simulink model "hpt_dual_dcpool_sw"  (R2025a)
settings: Solver=ode23tb  StartTime=0.0  StopTime=0.5  RelTol=1e-3
libraries: spsSeriesRLCBranchLib x5, spsControlledCurrentSourceLib x2, spsThreePhaseSeriesRLCBranchLib x2, spsThreePhaseVIMeasurementLib x2, spsVoltageMeasurementLib x2, spsUniversalBridgeLib x2, spsThreePhaseSourceLib x2, spsGroundLib x1, spsCurrentMeasurementLib x1, spspowerguiLib x1
settings Model: Creator=m1391  LastModifiedBy=m1391

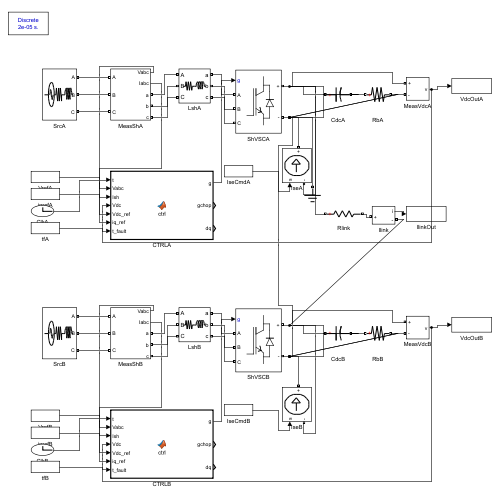
[thumbnail: Simulink's stored preview of the top-level diagram]
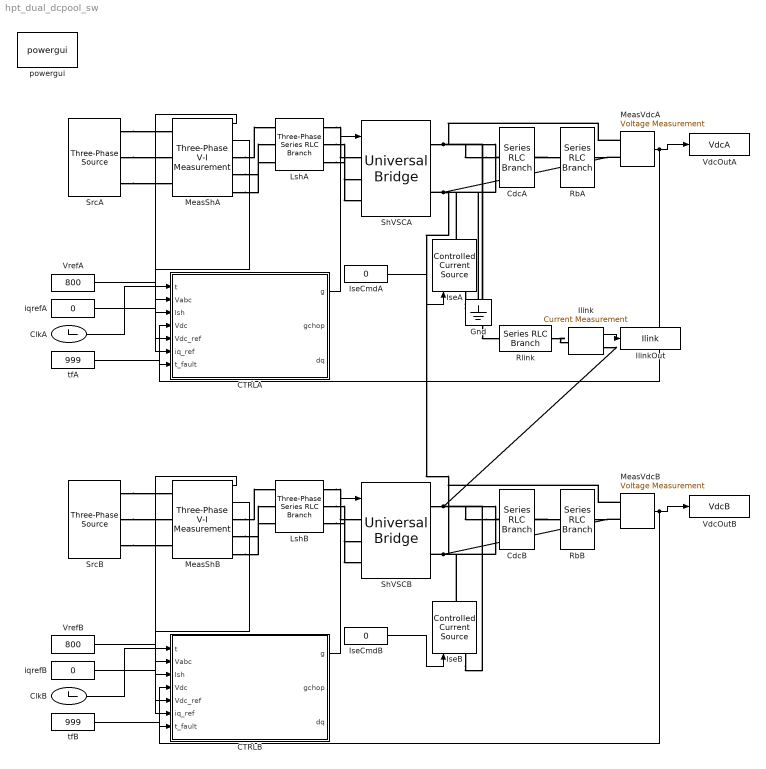
== system hpt_dual_dcpool_sw ==
  CTRLA : MATLAB Function  TreatAsAtomicUnit=on
  CTRLB : MATLAB Function  TreatAsAtomicUnit=on
  CdcA : spsSeriesRLCBranchLib/Series RLC Branch  LConnTagsString=__new0  RConnTagsString=__new0  BranchType=C  Resistance=1  Inductance=1e-3  SetiL0=off  InitialCurrent=0  Capacitance=0.0022  Setx0=on  InitialVoltage=800  Measurements=None
  CdcB : spsSeriesRLCBranchLib/Series RLC Branch  LConnTagsString=__new0  RConnTagsString=__new0  BranchType=C  Resistance=1  Inductance=1e-3  SetiL0=off  InitialCurrent=0  Capacitance=0.0022  Setx0=on  InitialVoltage=800  Measurements=None
  ClkA : Clock
  ClkB : Clock
  Gnd : spsGroundLib/Ground  LConnTagsString=a
  Ilink : spsCurrentMeasurementLib/Current Measurement  PhasorSimulation=off  OutputType=Complex  PSBequivalent=0
  IlinkOut : ToWorkspace  VariableName=Ilink  SampleTime=2e-05
  IseA : spsControlledCurrentSourceLib/Controlled Current Source  Initialize=on  Source_Type=AC  Amplitude=0  Phase=0  Frequency=0  Measurements=None
  IseB : spsControlledCurrentSourceLib/Controlled Current Source  Initialize=on  Source_Type=AC  Amplitude=0  Phase=0  Frequency=0  Measurements=None
  IseCmdA : Constant  Value=0
  IseCmdB : Constant  Value=0
  LshA : spsThreePhaseSeriesRLCBranchLib/Three-Phase Series RLC Branch  LConnTagsString=A|B|C  RConnTagsString=A|B|C  BranchType=RL  Resistance=0.05  Inductance=0.003  Capacitance=1e-6  Measurements=None
  LshB : spsThreePhaseSeriesRLCBranchLib/Three-Phase Series RLC Branch  LConnTagsString=A|B|C  RConnTagsString=A|B|C  BranchType=RL  Resistance=0.05  Inductance=0.003  Capacitance=1e-6  Measurements=None
  MeasShA : spsThreePhaseVIMeasurementLib/Three-Phase V-I Measurement  VoltageMeasurement=phase-to-ground  SetLabelV=off  LabelV=Vabc  Vpu=off  VpuLL=off  CurrentMeasurement=yes  SetLabelI=off  LabelI=Iabc  Ipu=off  Pbase=100e6  Vbase=500e3  OutputType=Complex  PhasorSimulation=off  PSBequivalent=0
  MeasShB : spsThreePhaseVIMeasurementLib/Three-Phase V-I Measurement  VoltageMeasurement=phase-to-ground  SetLabelV=off  LabelV=Vabc  Vpu=off  VpuLL=off  CurrentMeasurement=yes  SetLabelI=off  LabelI=Iabc  Ipu=off  Pbase=100e6  Vbase=500e3  OutputType=Complex  PhasorSimulation=off  PSBequivalent=0
  MeasVdcA : spsVoltageMeasurementLib/Voltage Measurement  PhasorSimulation=off  OutputType=Complex  PSBequivalent=0
  MeasVdcB : spsVoltageMeasurementLib/Voltage Measurement  PhasorSimulation=off  OutputType=Complex  PSBequivalent=0
  RbA : spsSeriesRLCBranchLib/Series RLC Branch  LConnTagsString=__new0  RConnTagsString=__new0  BranchType=R  Resistance=1e4  Inductance=1e-3  SetiL0=off  InitialCurrent=0  Capacitance=1e-6  Setx0=off  InitialVoltage=0  Measurements=None
  RbB : spsSeriesRLCBranchLib/Series RLC Branch  LConnTagsString=__new0  RConnTagsString=__new0  BranchType=R  Resistance=1e4  Inductance=1e-3  SetiL0=off  InitialCurrent=0  Capacitance=1e-6  Setx0=off  InitialVoltage=0  Measurements=None
  Rlink : spsSeriesRLCBranchLib/Series RLC Branch  LConnTagsString=__new0  RConnTagsString=__new0  BranchType=R  Resistance=0.5  Inductance=1e-3  SetiL0=off  InitialCurrent=0  Capacitance=1e-6  Setx0=off  InitialVoltage=0  Measurements=None
  ShVSCA : spsUniversalBridgeLib/Universal Bridge  Arms=3  SnubberResistance=1e5  SnubberCapacitance=inf  Device=IGBT / Diodes  Ron=1e-3  Lon=0  ForwardVoltages="[  0  0  ]"  ForwardVoltage=0  GTOparameters=[ 10e-6 , 20e-6 ]  IGBTparameters=[ 1e-6 , 2e-6 ]  Measurements=None  Measurements_2=None  converterType=Rectifier
  ShVSCB : spsUniversalBridgeLib/Universal Bridge  Arms=3  SnubberResistance=1e5  SnubberCapacitance=inf  Device=IGBT / Diodes  Ron=1e-3  Lon=0  ForwardVoltages="[  0  0  ]"  ForwardVoltage=0  GTOparameters=[ 10e-6 , 20e-6 ]  IGBTparameters=[ 1e-6 , 2e-6 ]  Measurements=None  Measurements_2=None  converterType=Rectifier
  SrcA : spsThreePhaseSourceLib/Three-Phase Source  InternalConnection=Y  VoltagePhases=off  Voltage=400  PhaseAngle=0  Voltage_phases=[25e3 25e3 25e3]/sqrt(3)  PhaseAngles_phases=[0 -120 +120]  Frequency=50  NonIdealSource=on  SpecifyImpedance=off  Resistance=1e-3  Inductance=1e-5  ShortCircuitLevel=100e6  BaseVoltage=25e3  XRratio=7  BusType=swing  Pref=10e3  Qref=0  Prefabc=[10e3, 10e3, 10e3]  Qrefabc=[0, 0, 0]  Qmin=-inf  Qmax=inf
  SrcB : spsThreePhaseSourceLib/Three-Phase Source  InternalConnection=Y  VoltagePhases=off  Voltage=400  PhaseAngle=0  Voltage_phases=[25e3 25e3 25e3]/sqrt(3)  PhaseAngles_phases=[0 -120 +120]  Frequency=50  NonIdealSource=on  SpecifyImpedance=off  Resistance=1e-3  Inductance=1e-5  ShortCircuitLevel=100e6  BaseVoltage=25e3  XRratio=7  BusType=swing  Pref=10e3  Qref=0  Prefabc=[10e3, 10e3, 10e3]  Qrefabc=[0, 0, 0]  Qmin=-inf  Qmax=inf
  VdcOutA : ToWorkspace  VariableName=VdcA  SampleTime=2e-05
  VdcOutB : ToWorkspace  VariableName=VdcB  SampleTime=2e-05
  VrefA : Constant  Value=800
  VrefB : Constant  Value=800
  iqrefA : Constant  Value=0
  iqrefB : Constant  Value=0
  powergui : spspowerguiLib/powergui  Priority=1  SimulationMode=Discrete  SampleTime=2e-05  frequency=60  Iterations=50  frequencyindice=60  Pbase=100e6  ErrMax=1e-4  UnitsV=kV  UnitsW=MW  buscounter=0  FunctionMessages=off  echomessages=off  EnableUseOfTLC=off  CurrentSourceSwitches=off  DisableSnubberDevices=off  DisableRonSwitches=off  DisableVfSwitches=off  DisplayEquations=off  AutomaticDiscreteSolvers=off  SolverType=Tustin/Backward Euler (TBE)  Interpol=off  ExternalGateDelay=off  methode=off  Ts=100  x0status=blocks  SPID=on  SwTol=0  HookPort=off  NonlinearTolerance=1e-4  nMaxIteration=100  ContinueOnMaxIteration=off  RestoreLinks=warning  ResistiveCurrentMeasurement=off  Frange=[0:2:500]  Ylog=off  Xlog=on  ShowGrid=off  save=off  variable=ZData  structure=0  ZoomFFT=off  StartTime=0.0  cycles=1  DisplayStyle=1  fundamental=60  FreqAxis=off  MaxFrequency=1000  frequencyindicesteady=1  RmsSteady=1  display=off
  tfA : Constant  Value=999
  tfB : Constant  Value=999
  wires:
  ClkA/1 -> CTRLA/1(t)
  MeasShA/1 -> CTRLA/2(Vabc)
  MeasShA/2 -> CTRLA/3(Ish)
  MeasVdcA/1 -> CTRLA/4(Vdc), VdcOutA/1
  VrefA/1 -> CTRLA/5(Vdc_ref)
  iqrefA/1 -> CTRLA/6(iq_ref)
  tfA/1 -> CTRLA/7(t_fault)
  CTRLA/1(g) -> ShVSCA/1
  IseCmdA/1 -> IseA/1
  ClkB/1 -> CTRLB/1(t)
  MeasShB/1 -> CTRLB/2(Vabc)
  MeasShB/2 -> CTRLB/3(Ish)
  MeasVdcB/1 -> CTRLB/4(Vdc), VdcOutB/1
  VrefB/1 -> CTRLB/5(Vdc_ref)
  iqrefB/1 -> CTRLB/6(iq_ref)
  tfB/1 -> CTRLB/7(t_fault)
  CTRLB/1(g) -> ShVSCB/1
  IseCmdB/1 -> IseB/1
  Ilink/1 -> IlinkOut/1
  connections:
  SrcA/RConn1 -- MeasShA/LConn1
  MeasShA/RConn1 -- LshA/LConn1
  LshA/RConn1 -- ShVSCA/LConn1
  SrcA/RConn2 -- MeasShA/LConn2
  MeasShA/RConn2 -- LshA/LConn2
  LshA/RConn2 -- ShVSCA/LConn2
  SrcA/RConn3 -- MeasShA/LConn3
  MeasShA/RConn3 -- LshA/LConn3
  LshA/RConn3 -- ShVSCA/LConn3
  CdcA/LConn1 -- ShVSCA/RConn1 -- RbA/LConn1 -- IseA/LConn1 -- MeasVdcA/LConn1 -- Rlink/LConn1
  SrcB/RConn1 -- MeasShB/LConn1
  MeasShB/RConn1 -- LshB/LConn1
  LshB/RConn1 -- ShVSCB/LConn1
  SrcB/RConn2 -- MeasShB/LConn2
  MeasShB/RConn2 -- LshB/LConn2
  LshB/RConn2 -- ShVSCB/LConn2
  SrcB/RConn3 -- MeasShB/LConn3
  MeasShB/RConn3 -- LshB/LConn3
  LshB/RConn3 -- ShVSCB/LConn3
  CdcB/LConn1 -- ShVSCB/RConn1 -- RbB/LConn1 -- IseB/LConn1 -- MeasVdcB/LConn1 -- Ilink/RConn1
  CdcB/RConn1 -- RbB/RConn1 -- IseB/RConn1 -- MeasVdcB/LConn2 -- ShVSCB/RConn2 -- CdcA/RConn1 -- RbA/RConn1 -- IseA/RConn1 -- MeasVdcA/LConn2 -- ShVSCA/RConn2 -- Gnd/LConn1
  Rlink/RConn1 -- Ilink/LConn1

== matlab function hpt_dual_dcpool_sw/CTRLB ==
  data: t input; g output; Vabc input; Ish input; Vdc input; Vdc_ref input; iq_ref input; t_fault input; gchop output; dq output
function [g, gchop, dq] = ctrl(t, Vabc, Ish, Vdc, Vdc_ref, iq_ref, t_fault)
%#codegen
persistent th wint idi iqi vdi tprev en idr
if isempty(th) || t < 1e-9
    th=0; wint=0; idi=0; iqi=0; vdi=0; tprev=0; en=0; idr=0;
end
if t > 0.15; en = 1; end
dt = t - tprev; if dt<0; dt=0; end; if dt>1e-3; dt=1e-3; end; tprev=t;
w0 = 2*pi*50; Lsh = 3e-3; Imax = 173.2;
Va=Vabc(1); Vb=Vabc(2); Vc=Vabc(3);
Valpha=(2/3)*(Va-0.5*Vb-0.5*Vc); Vbeta=(2/3)*(sqrt(3)/2)*(Vb-Vc);
Vd =  cos(th)*Valpha + sin(th)*Vbeta;
Vq = -sin(th)*Valpha + cos(th)*Vbeta;
Vm = sqrt(Vd*Vd+Vq*Vq); if Vm<100; Vm=100; end
err = Vq/Vm;
Kp_pll=90; Ki_pll=1500;
wint = wint + Ki_pll*err*dt; if wint>150; wint=150; elseif wint<-150; wint=-150; end
w = w0 + Kp_pll*err + wint; th = th + w*dt; th = mod(th,2*pi);
Ia=Ish(1); Ib=Ish(2); Ic=Ish(3);
Ialpha=(2/3)*(Ia-0.5*Ib-0.5*Ic); Ibeta=(2/3)*(sqrt(3)/2)*(Ib-Ic);
id =  cos(th)*Ialpha + sin(th)*Ibeta;
iq = -sin(th)*Ialpha + cos(th)*Ibeta;
Kpv=0.50; Kiv=8.0; ev=(Vdc_ref-Vdc)/Vdc_ref;
vdi = vdi + Kiv*ev*dt; if vdi>1; vdi=1; elseif vdi<-1; vdi=-1; end
idtgt=(Kpv*ev+vdi)*Imax; if idtgt>0.9*Imax; idtgt=0.9*Imax; elseif idtgt<-0.9*Imax; idtgt=-0.9*Imax; end
dmax=4000*dt; ds=idtgt-idr; if ds>dmax; ds=dmax; elseif ds<-dmax; ds=-dmax; end; idr=idr+ds;
iqr=iq_ref; if iqr>0.3*Imax; iqr=0.3*Imax; elseif iqr<-0.3*Imax; iqr=-0.3*Imax; end
idm=sqrt(max(0,Imax*Imax-iqr*iqr)); if idr<-idm; idr=-idm; elseif idr>idm; idr=idm; end
Kp=2.5; Ki=150; ed=idr-id; eq=iqr-iq;
ud = Vd-(Kp*ed+idi)+w0*Lsh*iq;
uq = Vq-(Kp*eq+iqi)-w0*Lsh*id;
half=max(50,Vdc/2); md=ud/half; mq=uq/half;
ma=md*cos(th)-mq*sin(th); mb=md*cos(th-2*pi/3)-mq*sin(th-2*pi/3); mc=md*cos(th+2*pi/3)-mq*sin(th+2*pi/3);
if ma>1; ma=1; elseif ma<-1; ma=-1; end
if mb>1; mb=1; elseif mb<-1; mb=-1; end
if mc>1; mc=1; elseif mc<-1; mc=-1; end
fc=5000; carrier=2*abs(2*(fc*t-floor(fc*t+0.5)))-1;
ga=ma>=carrier; gb=mb>=carrier; gc=mc>=carrier;
g=double([ga;~ga;gb;~gb;gc;~gc]);
if en<0.5; g=zeros(6,1); idi=0; iqi=0; vdi=0; end
sat=(abs(md)>1)||(abs(mq)>1);
if ~sat; idi=idi+Ki*ed*dt; iqi=iqi+Ki*eq*dt; if idi>300;idi=300;elseif idi<-300;idi=-300;end; if iqi>300;iqi=300;elseif iqi<-300;iqi=-300;end; end
gchop = double(Vdc > 1.20*800);
dq = [id; iq; idr; iqr; Vd; Vm; th];

== matlab function hpt_dual_dcpool_sw/CTRLA ==
  data: t input; g output; Vabc input; Ish input; Vdc input; Vdc_ref input; iq_ref input; t_fault input; gchop output; dq output
function [g, gchop, dq] = ctrl(t, Vabc, Ish, Vdc, Vdc_ref, iq_ref, t_fault)
%#codegen
persistent th wint idi iqi vdi tprev en idr
if isempty(th) || t < 1e-9
    th=0; wint=0; idi=0; iqi=0; vdi=0; tprev=0; en=0; idr=0;
end
if t > 0.15; en = 1; end
dt = t - tprev; if dt<0; dt=0; end; if dt>1e-3; dt=1e-3; end; tprev=t;
w0 = 2*pi*50; Lsh = 3e-3; Imax = 173.2;
Va=Vabc(1); Vb=Vabc(2); Vc=Vabc(3);
Valpha=(2/3)*(Va-0.5*Vb-0.5*Vc); Vbeta=(2/3)*(sqrt(3)/2)*(Vb-Vc);
Vd =  cos(th)*Valpha + sin(th)*Vbeta;
Vq = -sin(th)*Valpha + cos(th)*Vbeta;
Vm = sqrt(Vd*Vd+Vq*Vq); if Vm<100; Vm=100; end
err = Vq/Vm;
Kp_pll=90; Ki_pll=1500;
wint = wint + Ki_pll*err*dt; if wint>150; wint=150; elseif wint<-150; wint=-150; end
w = w0 + Kp_pll*err + wint; th = th + w*dt; th = mod(th,2*pi);
Ia=Ish(1); Ib=Ish(2); Ic=Ish(3);
Ialpha=(2/3)*(Ia-0.5*Ib-0.5*Ic); Ibeta=(2/3)*(sqrt(3)/2)*(Ib-Ic);
id =  cos(th)*Ialpha + sin(th)*Ibeta;
iq = -sin(th)*Ialpha + cos(th)*Ibeta;
Kpv=0.50; Kiv=8.0; ev=(Vdc_ref-Vdc)/Vdc_ref;
vdi = vdi + Kiv*ev*dt; if vdi>1; vdi=1; elseif vdi<-1; vdi=-1; end
idtgt=(Kpv*ev+vdi)*Imax; if idtgt>0.9*Imax; idtgt=0.9*Imax; elseif idtgt<-0.9*Imax; idtgt=-0.9*Imax; end
dmax=4000*dt; ds=idtgt-idr; if ds>dmax; ds=dmax; elseif ds<-dmax; ds=-dmax; end; idr=idr+ds;
iqr=iq_ref; if iqr>0.3*Imax; iqr=0.3*Imax; elseif iqr<-0.3*Imax; iqr=-0.3*Imax; end
idm=sqrt(max(0,Imax*Imax-iqr*iqr)); if idr<-idm; idr=-idm; elseif idr>idm; idr=idm; end
Kp=2.5; Ki=150; ed=idr-id; eq=iqr-iq;
ud = Vd-(Kp*ed+idi)+w0*Lsh*iq;
uq = Vq-(Kp*eq+iqi)-w0*Lsh*id;
half=max(50,Vdc/2); md=ud/half; mq=uq/half;
ma=md*cos(th)-mq*sin(th); mb=md*cos(th-2*pi/3)-mq*sin(th-2*pi/3); mc=md*cos(th+2*pi/3)-mq*sin(th+2*pi/3);
if ma>1; ma=1; elseif ma<-1; ma=-1; end
if mb>1; mb=1; elseif mb<-1; mb=-1; end
if mc>1; mc=1; elseif mc<-1; mc=-1; end
fc=5000; carrier=2*abs(2*(fc*t-floor(fc*t+0.5)))-1;
ga=ma>=carrier; gb=mb>=carrier; gc=mc>=carrier;
g=double([ga;~ga;gb;~gb;gc;~gc]);
if en<0.5; g=zeros(6,1); idi=0; iqi=0; vdi=0; end
sat=(abs(md)>1)||(abs(mq)>1);
if ~sat; idi=idi+Ki*ed*dt; iqi=iqi+Ki*eq*dt; if idi>300;idi=300;elseif idi<-300;idi=-300;end; if iqi>300;iqi=300;elseif iqi<-300;iqi=-300;end; end
gchop = double(Vdc > 1.20*800);
dq = [id; iq; idr; iqr; Vd; Vm; th];
